simulink library "lib_derating_reference_speed_limiter"  (R2023a)
settings: Solver=VariableStepAuto  StartTime=0.0  StopTime=10.0  RelTol=1e-3
libraries: lib_conversion x4, simulink x3, lib_discrete_time_integrator x1
settings Model: Creator=CAV2OFO  LastModifiedBy=lenovo
settings OptimizationCC: ReuseModelBlockBuffer=off

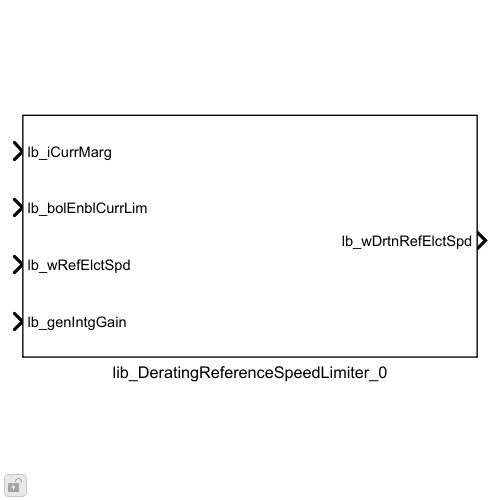
[thumbnail: Simulink's stored preview of the top-level diagram]
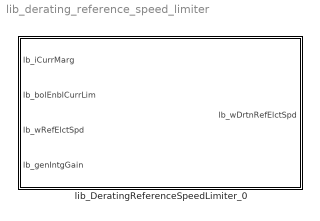
== system lib_derating_reference_speed_limiter ==
  lib_DeratingReferenceSpeedLimiter_0 : Subsystem  mask{lb_parSampTime=0.01, lb_parMaxSampTime=0.01, lb_parMaxIntgGain=1000, lb_parMaxCurrMarg=100, lb_parMinCurrMarg=-1, lb_parMaxElctRefSpd=2600, lb_parIntgScopMode=Integral control, lb_parSatFlag=on, lb_parAccmDataTypeMode=16-bit, lb_parDtiAccmDataTypeMode=Same of output, lb_parRefSpdDataType=fixdt(1,16,2^-3,0)}
      mask prompts: lb_parSampTime "Sampling time [s]:"; lb_parMaxSampTime "Maximum sampling time [s]:"; lb_parMaxIntgGain "Maximum integral gain [Nm*s/A]:"; lb_parMaxCurrMarg "Maximum current margin [A]:"; lb_parMinCurrMarg "Minimum current margin [A]:"; lb_parMaxElctRefSpd "Maximum reference speed [rad/s]:"; lb_parIntgScopMode "Integration scope:"; lb_parSatFlag "Output saturation"; lb_parAccmDataTypeMode "Accumulator data type mode:"; lb_parDtiAccmDataTypeMode "DTI accumulator data type mode:"; lb_parRefSpdDataType "DTI Output data type:"
      mask init:
      | lb_parMaxSampTime = double(lb_parSampTime);
      | lb_parMinCurrMarg = -double(lb_parMaxCurrMarg);
      | 
      | %% Req. XXX_030 - Define data type for internal reference speed
      | lb_parRefSpdDataType = Simulink.NumericType;
      | lb_parRefSpdDataType.DataTypeMode = 'Fixed-point: slope and bias scaling';
      | lb_parRefSpdDataType.Signedness = 'Signed';
      | switch lb_parAccmDataTypeMode
      |     case '16-bit'
      |         lb_parRefSpdDataType.WordLength = 16;
      |         temp.dataType = fi(lb_parMaxElctRefSpd);
      |         lb_parRefSpdDataType.Slope = 2^(-temp.dataType.FractionLength);
      |     case '32-bit'
      |         lb_parRefSpdDataType.WordLength = 32;
      |         temp.dataType = fi(lb_parMaxElctRefSpd,1,32);
      |         lb_parRefSpdDataType.Slope = 2^(-temp.dataType.FractionLength);
      | end
      | 
      | clear temp
      mask TypeOptions lb_parMaxSampTime: lib_DiscreteTimeIntegrator_1/lb_parMaxSampTime
      mask TypeOptions lb_parMaxIntgGain: lib_DiscreteTimeIntegrator_1/lb_parMaxIntgGain
      mask TypeOptions lb_parMaxCurrMarg: lib_DiscreteTimeIntegrator_1/lb_parMaxInpVal
      mask TypeOptions lb_parMinCurrMarg: lib_DiscreteTimeIntegrator_1/lb_parMinInpVal
      mask TypeOptions lb_parIntgScopMode: lib_DiscreteTimeIntegrator_1/lb_parIntgScopMode
      mask TypeOptions lb_parSatFlag: lib_DiscreteTimeIntegrator_1/lb_parSatFlag
      mask TypeOptions lb_parAccmDataTypeMode: 16-bit | 32-bit
      mask TypeOptions lb_parDtiAccmDataTypeMode: lib_DiscreteTimeIntegrator_1/lb_parAccmDataTypeMode
      mask TypeOptions lb_parRefSpdDataType: lib_DiscreteTimeIntegrator_1/lb_parOutpDataType
      mask DialogControl Container2 Prompt: VHIT control library
      mask DialogControl Control1 Prompt: Derating reference speed limiter
      mask DialogControl Container1 Prompt: Parameters
      mask DialogControl Container3 Prompt: Operating modes:
      mask DialogControl Container4 Prompt: Data types

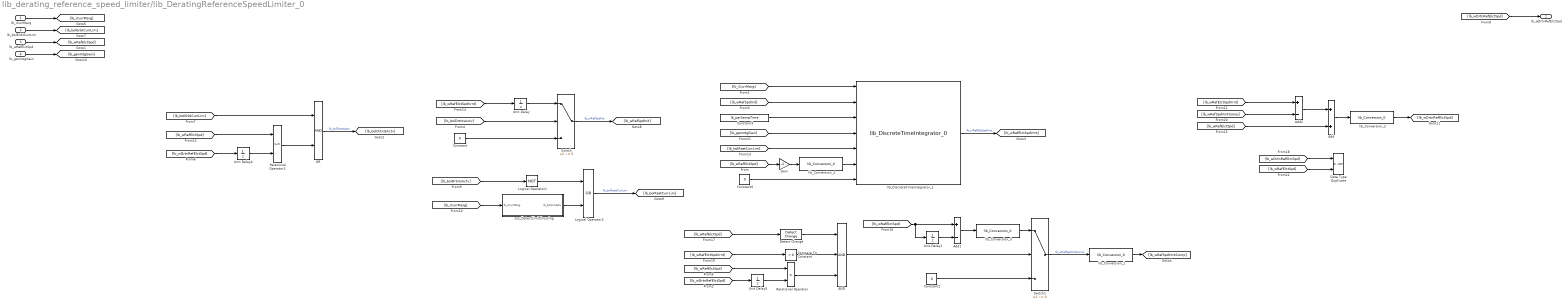
== system lib_derating_reference_speed_limiter/lib_DeratingReferenceSpeedLimiter_0 ==
  lb_iCurrMarg : Inport  OutMin=-lb_parMaxCurrMarg  OutMax=lb_parMaxCurrMarg
  lb_bolEnblCurrLim : Inport  Port=2  OutDataTypeStr=boolean
  lb_wRefElctSpd : Inport  Port=3  OutMin=0  OutMax=lb_parMaxElctRefSpd
  lb_genIntgGain : Inport  Port=4  OutMin=0  OutMax=lb_parMaxIntgGain
  AND : Logic  Inputs=3  AllPortsSameDT=off  OutDataTypeStr=boolean
  Add : Sum  OutDataTypeStr=Inherit: Inherit via back propagation
  Add1 : Sum  Inputs=+-  OutDataTypeStr=Inherit: Inherit via back propagation
  Add2 : Sum  Inputs=+-  OutDataTypeStr=Inherit: Same as first input
  Compare To Constant : simulink/Logic and Bit Operations/Compare To Constant  relop=<  const=0  OutDataTypeStr=boolean
  Constant : Constant  Value=0  OutDataTypeStr=lb_parRefSpdDataType
  Constant1 : Constant  Value=0  OutDataTypeStr=lb_parRefSpdDataType
  Constant3 : Constant  Value=lb_parSampTime
  Constant5 : Constant  Value=0  OutDataTypeStr=lb_parRefSpdDataType
  Data Type Duplicate : DataTypeDuplicate
  Detect Change : simulink/Logic and Bit Operations/Detect Change  vinit=0  OutDataTypeStr=boolean
  Gain : Gain  Gain=-1  OutDataTypeStr=Inherit: Inherit via back propagation
  Logical Operator1 : Logic  Operator=NOT  AllPortsSameDT=off  OutDataTypeStr=boolean
  Logical Operator2 : Logic  Operator=OR  AllPortsSameDT=off  OutDataTypeStr=boolean
  OR : Logic  AllPortsSameDT=off  OutDataTypeStr=boolean
  Relational Operator : RelationalOperator  Operator=>  OutDataTypeStr=boolean  RndMeth=Simplest  InputSameDT=off
  Relational Operator1 : RelationalOperator  OutDataTypeStr=boolean  RndMeth=Simplest  InputSameDT=off
  Switch : Switch  Criteria=u2 ~= 0  SaturateOnIntegerOverflow=off  InputSameDT=off
  Switch1 : Switch  Criteria=u2 ~= 0  SaturateOnIntegerOverflow=off  InputSameDT=off
  Unit Delay{,1,3..4} (4 alike) : UnitDelay  SampleTime=-1  HasFrameUpgradeWarning=on
  lib_Conversion_1 : lib_conversion/lib_Conversion_0  lb_parDataType=lb_parRefSpdDataType  lb_parOutpMaxVal=[]  lb_parOutpMinVal=[]  lb_parSatFlag=off
  lib_Conversion_2 : lib_conversion/lib_Conversion_0  lb_parDataType=Inherit: Inherit via back propagation  lb_parOutpMaxVal=[]  lb_parOutpMinVal=[]  lb_parSatFlag=off
  lib_Conversion_3 : lib_conversion/lib_Conversion_0  lb_parDataType=lb_parRefSpdDataType  lb_parOutpMaxVal=[]  lb_parOutpMinVal=[]  lb_parSatFlag=off
  lib_Conversion_4 : lib_conversion/lib_Conversion_0  lb_parDataType=lb_parRefSpdDataType  lb_parOutpMaxVal=[]  lb_parOutpMinVal=[]  lb_parSatFlag=off
  lib_DiscreteTimeIntegrator_1 : lib_discrete_time_integrator/lib_DiscreteTimeIntegrator_0  lb_parMaxInpVal=lb_parMaxCurrMarg  lb_parMinInpVal=lb_parMinCurrMarg  lb_parMaxSampTime=lb_parMaxSampTime  lb_parMaxIntgGain=lb_parMaxIntgGain  lb_parAccmDataTypeMode=Same of output  lb_parOutpDataType=fixdt(1,16,2^-3,0)  lb_parIntgScopMode=Integral control  lb_parSatFlag=on
      settings: LibrarySourceBlock=vhit_control_library/lib_DiscreteTimeIntegrator_0
  sss_DetectLimitCrossing : Subsystem
  lb_wDrtnRefElctSpd : Outport
  wires:
  [lb_wRefElctSpdVrnt] -> Add2/1
  lib_DiscreteTimeIntegrator_1/1 -> [lb_wRefElctSpdVrnt]  "lb_wRefElctSpdVrnt"
  [lb_wRefElctSpd] -> Relational Operator/1
  Unit Delay/1 -> Switch/1
  [lb_wDrtnRefElctSpd] -> lb_wDrtnRefElctSpd/1
  [lb_wRefSpdInit] -> lib_DiscreteTimeIntegrator_1/2
  [lb_wRefElctSpd] -> Gain/1
  Constant5/1 -> lib_DiscreteTimeIntegrator_1/7
  lb_iCurrMarg/1 -> [lb_iCurrMarg]
  lb_wRefElctSpd/1 -> [lb_wRefElctSpd]
  lb_bolEnblCurrLim/1 -> [lb_bolEnblCurrLim]
  Switch/1 -> [lb_wRefSpdInit]  "lb_wRefSpdInit"
  [lb_bolDrtnIsActv] -> Switch/2
  Logical Operator1/1 -> Logical Operator2/1
  Logical Operator2/1 -> [lb_bolRsetCurrLim]  "lb_bolRsetCurrLim"
  [lb_wRefElctSpdVrnt] -> Unit Delay/1
  Constant/1 -> Switch/3
  [lb_iCurrMarg] -> sss_DetectLimitCrossing/1(lb_iCurrMarg)
  sss_DetectLimitCrossing/1(lb_bolLimActv) -> Logical Operator2/2
  [lb_iCurrMarg] -> lib_DiscreteTimeIntegrator_1/1
  [lb_bolRsetCurrLim] -> lib_DiscreteTimeIntegrator_1/5
  Constant3/1 -> lib_DiscreteTimeIntegrator_1/3
  [lb_genIntgGain] -> lib_DiscreteTimeIntegrator_1/4
  Unit Delay1/1 -> Add1/2
  Add2/1 -> Add/1
  Add1/1 -> lib_Conversion_3/1
  Detect Change/1 -> AND/1
  Constant1/1 -> Switch1/3
  Compare To Constant/1 -> AND/2
  AND/1 -> Switch1/2
  Relational Operator/1 -> AND/3
  Unit Delay3/1 -> Relational Operator/2
  [lb_wDrtnRefElctSpd] -> Unit Delay4/1
  [lb_wRefElctSpd] -> Relational Operator1/1
  [lb_bolEnblCurrLim] -> OR/1
  Unit Delay4/1 -> Relational Operator1/2
  Relational Operator1/1 -> OR/2
  OR/1 -> [lb_bolDrtnIsActv]  "lb_bolDrtnIsActv"
  [lb_bolDrtnIsActv] -> Logical Operator1/1
  [lb_wRefElctSpd] -> Add/2
  [lb_wRefElctSpd] -> Unit Delay1/1, Add1/1
  [lb_wRefElctSpd] -> Detect Change/1
  [lb_wDrtnRefElctSpd] -> Unit Delay3/1
  [lb_wRefElctSpdVrnt] -> Compare To Constant/1
  Switch1/1 -> lib_Conversion_1/1  "lb_wRefSpdVrntComp"
  [lb_wRefSpdVrntComp] -> Add2/2
  lb_genIntgGain/1 -> [lb_genIntgGain]
  lib_Conversion_1/1 -> [lb_wRefSpdVrntComp]
  lib_Conversion_2/1 -> [lb_wDrtnRefElctSpd]
  Add/1 -> lib_Conversion_2/1
  [lb_wDrtnRefElctSpd] -> Data Type Duplicate/1
  [lb_wRefElctSpd] -> Data Type Duplicate/2
  lib_Conversion_3/1 -> Switch1/1
  lib_Conversion_4/1 -> lib_DiscreteTimeIntegrator_1/6
  Gain/1 -> lib_Conversion_4/1

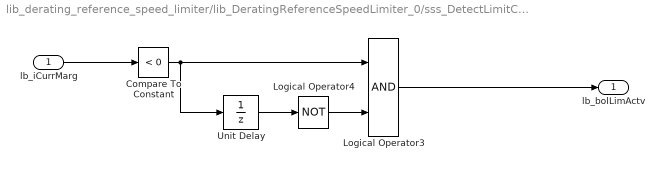
== system lib_derating_reference_speed_limiter/lib_DeratingReferenceSpeedLimiter_0/sss_DetectLimitCrossing ==
  lb_iCurrMarg : Inport
  Compare To Constant : simulink/Logic and Bit Operations/Compare To Constant  relop=<  const=0  OutDataTypeStr=boolean
  Logical Operator3 : Logic  AllPortsSameDT=off  OutDataTypeStr=boolean
  Logical Operator4 : Logic  Operator=NOT  AllPortsSameDT=off  OutDataTypeStr=boolean
  Unit Delay : UnitDelay  SampleTime=-1  HasFrameUpgradeWarning=on
  lb_bolLimActv : Outport
  wires:
  Logical Operator3/1 -> lb_bolLimActv/1
  lb_iCurrMarg/1 -> Compare To Constant/1
  Logical Operator4/1 -> Logical Operator3/2
  Unit Delay/1 -> Logical Operator4/1
  Compare To Constant/1 -> Unit Delay/1, Logical Operator3/1
